simulink model "recursive_running_sum"  (R2014b)
settings: Solver=ode45  StartTime=0.0  StopTime=inf  RelTol=1e-3
libraries: commchan3 x1
settings Model: Creator=Ben  LastModifiedBy=Ben

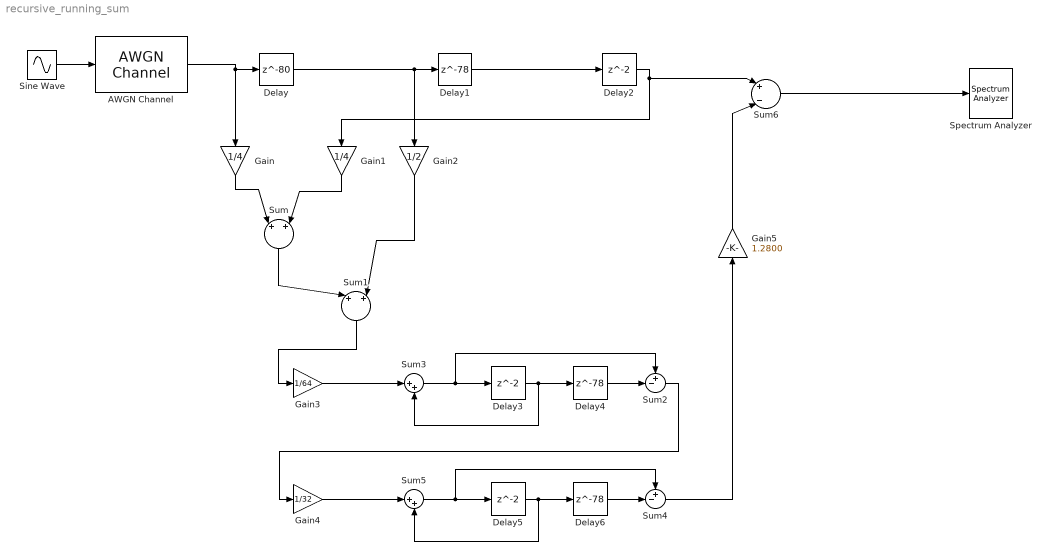
== system recursive_running_sum ==
  AWGN Channel : commchan3/AWGN Channel  InputProcessing=Columns as channels (frame based)  seed=67  noiseMode="Signal to noise ratio  (Eb/No)"  EbNodB=-50  EsNodB=10  SNRdB=10  bitsPerSym=1  Ps=1  Tsym=1  variance=1
  Delay : Delay  DelayLength=80  InitialCondition=0
  Delay1 : Delay  DelayLength=78  InitialCondition=0
  Delay2 : Delay  InitialCondition=0
  Delay3 : Delay  InitialCondition=0
  Delay4 : Delay  DelayLength=78  InitialCondition=0
  Delay5 : Delay  InitialCondition=0
  Delay6 : Delay  DelayLength=78  InitialCondition=0
  Gain : Gain  Gain=1/4
  Gain1 : Gain  Gain=1/4
  Gain2 : Gain  Gain=1/2
  Gain3 : Gain  Gain=1/64
  Gain4 : Gain  Gain=1/32
  Gain5 : Gain  Gain=1.2800
  Sine Wave : Sin  Frequency=23*2*pi  SampleTime=1/100
  Spectrum Analyzer : SpectrumAnalyzer
  Sum : Sum  Inputs=|+|+|
  Sum1 : Sum  Inputs=|+|+|
  Sum2 : Sum  Inputs=+-|
  Sum3 : Sum  Inputs=|++
  Sum4 : Sum  Inputs=+-|
  Sum5 : Sum  Inputs=|++
  Sum6 : Sum  Inputs=|+|-|
  wires:
  Sine Wave/1 -> AWGN Channel/1
  Delay/1 -> Gain2/1, Delay1/1
  Delay1/1 -> Delay2/1
  Gain1/1 -> Sum/2
  Gain/1 -> Sum/1
  Delay2/1 -> Sum6/1, Gain1/1
  Sum/1 -> Sum1/1
  Gain2/1 -> Sum1/2
  Sum1/1 -> Gain3/1
  Gain3/1 -> Sum3/1
  Sum3/1 -> Sum2/1, Delay3/1
  Delay3/1 -> Delay4/1, Sum3/2
  Delay4/1 -> Sum2/2
  Gain4/1 -> Sum5/1
  Sum5/1 -> Sum4/1, Delay5/1
  Delay5/1 -> Delay6/1, Sum5/2
  Delay6/1 -> Sum4/2
  Sum2/1 -> Gain4/1
  Sum4/1 -> Gain5/1
  Gain5/1 -> Sum6/2
  Sum6/1 -> Spectrum Analyzer/1
  AWGN Channel/1 -> Gain/1, Delay/1
